simulink model "adc_demo"  (Simulink 8.3)
settings: Solver=VariableStepDiscrete  StartTime=0.0  StopTime=1  RelTol=1e-3
libraries: simulink_extras x1
settings Model: Creator=rcheng  LastModifiedBy=rodralez
settings OptimizationCC: ExpressionDepthLimit=2147483647  InitFltsAndDblsToZero=on
settings DebuggingCC: FcnCallInpInsideContextMsg=UseLocalSettings

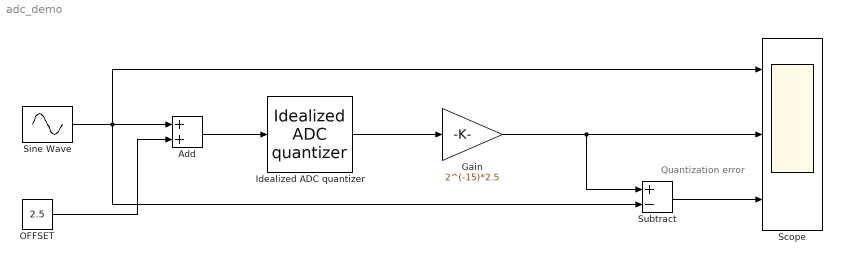
== system adc_demo ==
  note: Quantization error
  Add : Sum
  Gain : Gain  Gain=2^(-15)*2.5
  Idealized ADC quantizer : simulink_extras/Additional Discrete/Idealized ADC quantizer  NumberOfConverterBits=16  Vmin=0  Vmax=5  OutputDataType=int16  OutputNegativeValues=on
  OFFSET : Constant  Value=2.5
  Scope : Scope  NumInputPorts=3
      settings: ShowLegends=on  TimeRange=0.5  YMin=-5~-5~-5  YMax=5~5~5
  Sine Wave : Sin  Amplitude=2.5  Frequency=2*pi*100  SampleTime=1/10000
  Subtract : Sum  Inputs=+-
  wires:
  Subtract/1 -> Scope/3
  Sine Wave/1 -> Subtract/2, Scope/1, Add/1
  Add/1 -> Idealized ADC quantizer/1
  OFFSET/1 -> Add/2
  Idealized ADC quantizer/1 -> Gain/1
  Gain/1 -> Scope/2, Subtract/1
